simulink model "PitchPID"  (R2021a)
settings: Solver=VariableStepAuto  StartTime=0.0  StopTime=30  RelTol=1e-3
values from neighbouring files (symbols this model uses):
  body_pitch_b = 0.0015675980775375    (= 0.00156759807754)    [setup.m]
  body_pitch_m = -0.250343385330279    (= -0.25034338533)    [setup.m]
  elevator_m = 0.0842508724650606    (= 0.0842508724651)    [setup.m]
  I_yy = 1.711    [setup.m]
  initial_roll = asin(-body_pitch_b / body_pitch_m)    [setup.m]
  v = sqrt(mass * g / lift_b)    [setup.m]
libraries: simulink_extras x2, pid_lib x1
settings Model: Creator=corwi  LastModifiedBy=amaar
settings SolverCC: AlgebraicLoopSolver=TrustRegion
settings DebuggingCC: SFMachineParentedDataDiag=warning

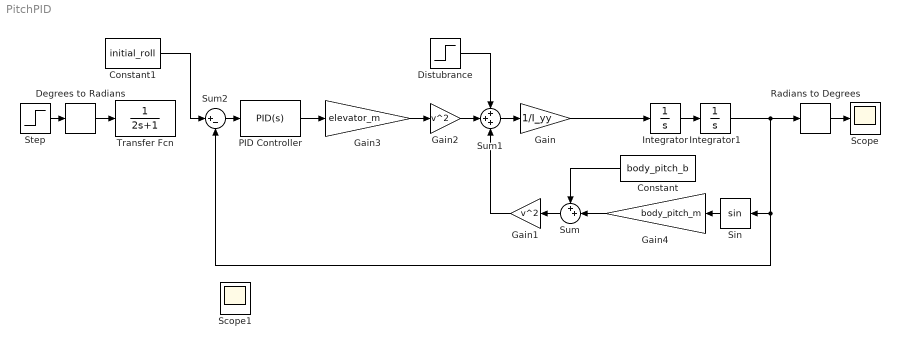
== system PitchPID ==
  Constant : Constant  Value=body_pitch_b
  Constant1 : Constant  Value=initial_roll
  Degrees to Radians : simulink_extras/Transformations/Degrees to Radians
  Distubrance : Step  Time=0  SampleTime=0
  Gain : Gain  Gain=1/I_yy
  Gain1 : Gain  Gain=v^2
  Gain2 : Gain  Gain=v^2
  Gain3 : Gain  Gain=elevator_m
  Gain4 : Gain  Gain=body_pitch_m
  Integrator : Integrator
  Integrator1 : Integrator  InitialCondition=initial_roll
  PID Controller : pid_lib/PID Controller  Controller=PID  Form=Parallel  TimeDomain=Continuous-time  UseExternalTs=off  SampleTime=-1  IntegratorMethod=Forward Euler  FilterMethod=Forward Euler  ControllerParametersSource=internal  P=35  I=15  D=10  UseFilter=on  N=100  TunerSelectOption=Transfer Function Based (PID Tuner App)  InitialConditionSource=internal  InitialConditionForIntegrator=0  InitialConditionForFilter=0  DifferentiatorICPrevScaledInput=0  ExternalReset=none  TrackingMode=off  Kt=1  LimitOutput=on  SatLimitsSource=internal  UpperSaturationLimit=6  LowerSaturationLimit=-pi/6  LinearizeAsGain=on  AntiWindupMode=none  Kb=1  POutMin=[]  POutMax=[]  IOutMin=[]  IOutMax=[]  DOutMin=[]  DOutMax=[]  NOutMin=[]  NOutMax=[]  SumOutMin=[]  SumOutMax=[]  SaturationOutMin=[]  SaturationOutMax=[]  PParamMin=[]  PParamMax=[]  IParamMin=[]  IParamMax=[]  DParamMin=[]  DParamMax=[]  NParamMin=[]  NParamMax=[]  KbParamMin=[]  KbParamMax=[]  KtParamMin=[]  KtParamMax=[]  KbOutMin=[]  KbOutMax=[]  KtOutMin=[]  KtOutMax=[]  IntegratorOutMin=[]  IntegratorOutMax=[]  FilterOutMin=[]  FilterOutMax=[]  SumI1OutMin=[]  SumI1OutMax=[]  SumI2OutMin=[]  SumI2OutMax=[]  SumI3OutMin=[]  SumI3OutMax=[]  SumI4OutMin=[]  SumI4OutMax=[]  SumDOutMin=[]  SumDOutMax=[]  DifferentiatorOutMin=[]  DifferentiatorOutMax=[]  FilterDiffOutCoefMin=[]  FilterDiffOutCoefMax=[]  ReciprocalOutMin=[]  ReciprocalOutMax=[]  SumDenOutMin=[]  SumDenOutMax=[]  SumNumOutMin=[]  SumNumOutMax=[]  DivideOutMin=[]  DivideOutMax=[]  UdiffTsProdOutMin=[]  UdiffTsProdOutMax=[]  NTsProdOutMin=[]  NTsProdOutMax=[]  UintegralTsProdOutMin=[]  UintegralTsProdOutMax=[]  UngainTsProdOutMin=[]  UngainTsProdOutMax=[]  IntegratorContinuousStateAttributes=''  IntegratorStateMustResolveToSignalObject=off  IntegratorRTWStateStorageClass=Auto  FilterContinuousStateAttributes=''  FilterStateMustResolveToSignalObject=off  FilterRTWStateStorageClass=Auto  ParallelPVariant=InternalParameters  IdealPVariant=Disabled  IVariant=InternalParameters  DVariant=InternalParameters  IntegratorVariant=Continuous  SatVariant=Enabled  AWVariant=Passthrough  PCopyVariant=Disabled  TRVariant=Disabled  FdbkBlocksVariant=Forward  IdealPFdbkVariant=Disabled  SatFdbkVariant=Disabled  DerivativeFilterVariant=ContFilter  NVariant=InternalParameters  NCopyVariant=Disabled  FilterICVariant=InternalICsFilter  IntegratorICVariant=InternalICs  ExternalResetVariant=Disabled  TRSumVariant=Passthrough  SumFdbkVariant=Disabled  SumVariant=Sum_PID  TsampFilterVariant=InternalTs  TsampNgainVariant=Passthrough  TsampIntegralVariant=Passthrough  ExternalSaturationOutDataTypeStr=Inherit: Same as second input
  Radians to Degrees : simulink_extras/Transformations/Radians to Degrees
  Scope : Scope
  Scope1 : Scope
  Sin : Trigonometry
  Step : Step  Time=0  After=0  SampleTime=0
  Sum : Sum  Inputs=++|
  Sum1 : Sum  Inputs=+++
  Sum2 : Sum  Inputs=|+-
  Transfer Fcn : TransferFcn  Denominator=[2 1]
  wires:
  Gain/1 -> Integrator/1
  Integrator/1 -> Integrator1/1
  Integrator1/1 -> Sum2/2, Sin/1, Radians to Degrees/1
  Sin/1 -> Gain4/1
  Constant/1 -> Sum/1
  Gain4/1 -> Sum/2
  Sum2/1 -> PID Controller/1
  Sum1/1 -> Gain/1
  Gain3/1 -> Gain2/1
  Radians to Degrees/1 -> Scope/1
  Step/1 -> Degrees to Radians/1
  Gain2/1 -> Sum1/2
  Distubrance/1 -> Sum1/1
  Sum/1 -> Gain1/1
  Gain1/1 -> Sum1/3
  PID Controller/1 -> Gain3/1
  Degrees to Radians/1 -> Transfer Fcn/1
  Constant1/1 -> Sum2/1
